simulink model "DC_motor_SMC_c"  (R2015b)
settings: Solver=VariableStepAuto  StartTime=0.0  StopTime=20  RelTol=1e-3
libraries: simulink x3
settings Model: Creator=mgreiff  LastModifiedBy=mgreiff
settings DebuggingCC: AlgebraicLoopMsg=none

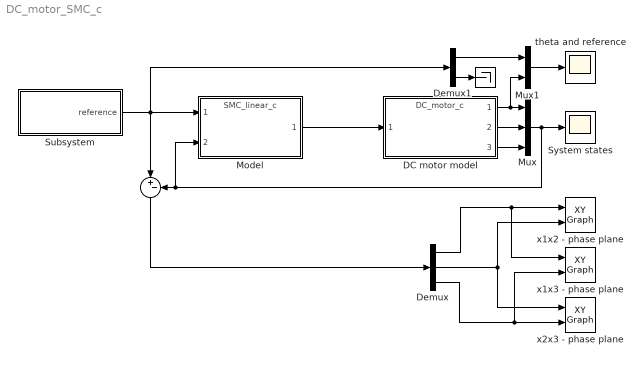
== system DC_motor_SMC_c ==
  " " : Sum  Inputs=|+-
  "    " : Terminator
  DC motor model : ModelReference  ModelNameDialog=DC_motor_c.slx  SimulationMode=Normal  ModelReferenceVersion=1.8  CopyOfModelName=DC_motor_c.slx
  Demux : Demux  Outputs=3
  Demux1 : Demux  Outputs=[1,2]
  Model : ModelReference  ModelNameDialog=SMC_linear_c.slx  SimulationMode=Normal  ModelReferenceVersion=1.2  CopyOfModelName=SMC_linear_c.slx
  Mux : Mux  Inputs=3
  Mux1 : Mux  Inputs=2
  Subsystem : Subsystem
  System states : Scope
  theta and reference : Scope
  x1x2 - phase plane : simulink/Sinks/XY Graph  xmin=-10  xmax=10  ymin=-10  ymax=10  st=-1
  x1x3 - phase plane : simulink/Sinks/XY Graph  xmin=-10  xmax=10  ymin=-10  ymax=10  st=-1
  x2x3 - phase plane : simulink/Sinks/XY Graph  xmin=-10  xmax=10  ymin=-10  ymax=10  st=-1
  wires:
  DC motor model/3 -> Mux/3
  DC motor model/1 -> Mux/1, Mux1/2
  DC motor model/2 -> Mux/2
  " "/1 -> Demux/1
  Demux/1 -> x1x3 - phase plane/1, x1x2 - phase plane/1
  Demux/2 -> x1x2 - phase plane/2, x2x3 - phase plane/1
  Demux/3 -> x1x3 - phase plane/2, x2x3 - phase plane/2
  Subsystem/1(reference) -> Model/1, Demux1/1, " "/1
  Mux1/1 -> theta and reference/1
  Demux1/1 -> Mux1/1
  Demux1/2 -> "    "/1
  Model/1 -> DC motor model/1
  Mux/1 -> Model/2, " "/2, System states/1

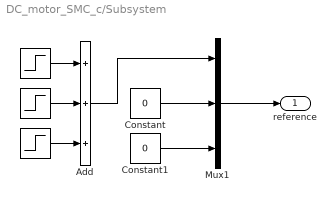
== system DC_motor_SMC_c/Subsystem ==
  " " : Step  Time=5  SampleTime=0
  "  " : Step  Time=10  After=-2  SampleTime=0
  "   " : Step  Time=15  After=1.5  SampleTime=0
  Add : Sum  Inputs=+++
  Constant : Constant  Value=0
  Constant1 : Constant  Value=0
  Mux1 : Mux  Inputs=3
  reference : Outport  PortDimensions=3
  wires:
  Add/1 -> Mux1/1
  Constant/1 -> Mux1/2
  Constant1/1 -> Mux1/3
  Mux1/1 -> reference/1
  " "/1 -> Add/1
  "  "/1 -> Add/2
  "   "/1 -> Add/3
